simulink model "desaturation"  (R2020b)
settings: Solver=ode15s  StartTime=27585  StopTime=44962.012  MaxStep=0.1  RelTol=1e-8  AbsTol=1e-8
values from neighbouring files (symbols this model uses):
  data = struct()    [config.m]    (also in config6U.m; configSlew.m; mainOffNominal.m = dataFix; statisticalAnalysis.m = dataFix)
undefined symbols (not defined in the file or in its folder): spacecraft
libraries: dspswit3 x1, simulink_extras x1
(part 1 of 2)
settings Model: SimulationMode=accelerator  Creator=pacif  LastModifiedBy=pacif

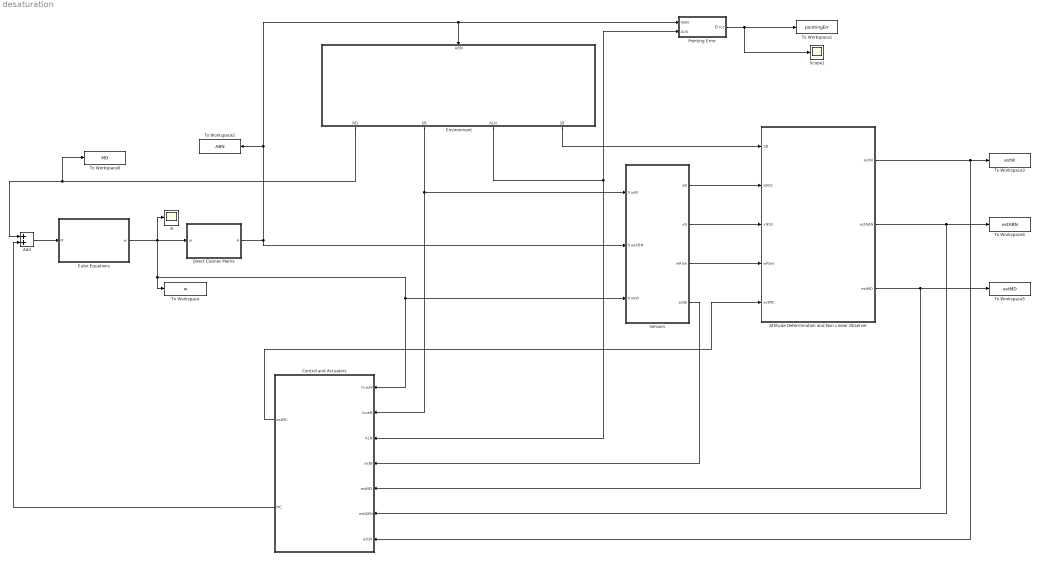
== system desaturation ==
  Add : Sum
  Attitude Determination and Non Linear Observer : Subsystem
  Control and Actuators : Subsystem
  Direct Cosines Matrix : Subsystem
  Environment : Subsystem
  Euler Equations : Subsystem
  Pointing Error : Subsystem
  Scope1 : Scope
  Sensors : Subsystem
  To Workspace : ToWorkspace  VariableName=w  SaveFormat=Timeseries  SampleTime=-1
  To Workspace1 : ToWorkspace  VariableName=pointingErr  SaveFormat=Timeseries  SampleTime=-1
  To Workspace2 : ToWorkspace  VariableName=ABN  SaveFormat=Timeseries  SampleTime=-1
  To Workspace3 : ToWorkspace  VariableName=estW  SaveFormat=Timeseries  SampleTime=-1
  To Workspace4 : ToWorkspace  VariableName=estABN  SaveFormat=Timeseries  SampleTime=-1
  To Workspace5 : ToWorkspace  VariableName=estMD  SaveFormat=Timeseries  SampleTime=-1
  To Workspace6 : ToWorkspace  VariableName=MD  SaveFormat=Timeseries  SampleTime=-1
  w : Scope
  wires:
  Environment/2(bB) -> Sensors/1(trueB), Control and Actuators/2(trueB)
  Add/1 -> Euler Equations/1(M)
  Environment/1(MD) -> To Workspace6/1, Add/1
  Euler Equations/1(w) -> Direct Cosines Matrix/1(w), To Workspace/1, Control and Actuators/1(trueW), Sensors/3(trueW), w/1
  Direct Cosines Matrix/1(A) -> To Workspace2/1, Environment/1(ABN), Pointing Error/1(ABN), Sensors/2(trueABN)
  Environment/3(ALN) -> Pointing Error/2(ALN), Control and Actuators/3(ALN)
  Control and Actuators/2(MC) -> Add/2
  Sensors/4(estB) -> Control and Actuators/4(estB)
  Control and Actuators/1(estMC) -> Attitude Determination and Non Linear Observer/5(estMC)
  Environment/4(SB) -> Attitude Determination and Non Linear Observer/1(SB)
  Attitude Determination and Non Linear Observer/2(estABN) -> Control and Actuators/6(estABN), To Workspace4/1
  Attitude Determination and Non Linear Observer/3(estMD) -> Control and Actuators/5(estMD), To Workspace5/1
  Pointing Error/1(Error) -> Scope1/1, To Workspace1/1
  Sensors/1(sB) -> Attitude Determination and Non Linear Observer/2(sBSS)
  Sensors/2(vN) -> Attitude Determination and Non Linear Observer/3(vNSS)
  Sensors/3(wRaw) -> Attitude Determination and Non Linear Observer/4(wRaw)
  Attitude Determination and Non Linear Observer/1(estW) -> Control and Actuators/7(estW), To Workspace3/1

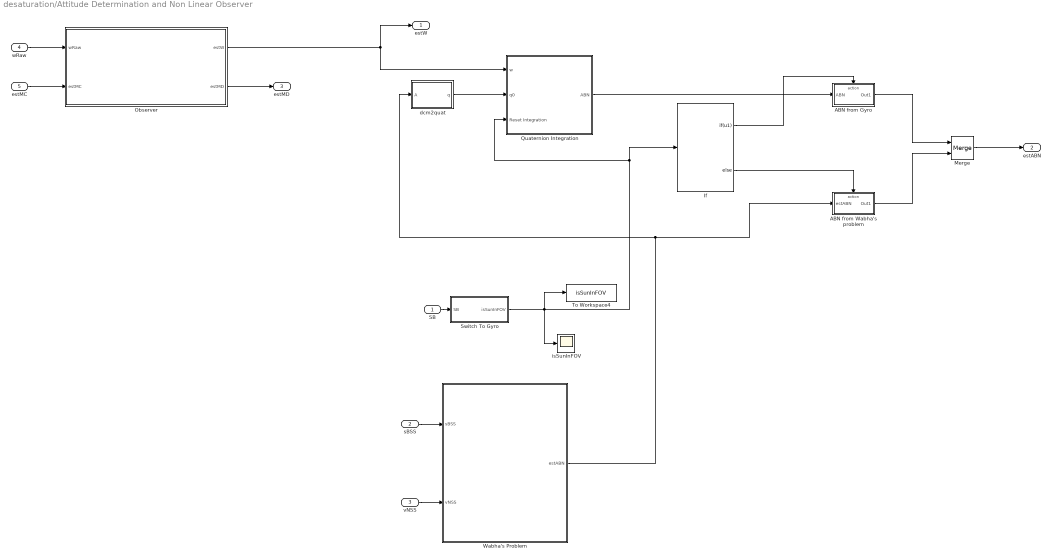
== system desaturation/Attitude Determination and Non Linear Observer ==
  SB : Inport
  sBSS : Inport  Port=2
  vNSS : Inport  Port=3
  wRaw : Inport  Port=4
  estMC : Inport  Port=5
  ABN from Gyro : Subsystem  TreatAsAtomicUnit=on
  ABN from Wabha's problem : Subsystem  TreatAsAtomicUnit=on
  If : If  IfExpression=u1
  Merge : Merge
  Observer : Subsystem
  "Quaternion Integration " : Subsystem
  Switch To Gyro : Subsystem
  To Workspace4 : ToWorkspace  VariableName=isSunInFOV  SaveFormat=Timeseries  SampleTime=-1
  Wabha's Problem : MATLAB Function  TreatAsAtomicUnit=on
  dcm2quat : MATLAB Function  TreatAsAtomicUnit=on
  isSunInFOV : Scope
  estW : Outport
  estABN : Outport  Port=2
  estMD : Outport  Port=3
  wires:
  wRaw/1 -> Observer/1(wRaw)
  SB/1 -> Switch To Gyro/1(SB)
  ABN from Wabha's problem/1(Out1) -> Merge/2
  Merge/1 -> estABN/1
  If/1 -> ABN from Gyro/Action
  If/2 -> ABN from Wabha's problem/Action
  ABN from Gyro/1(Out1) -> Merge/1
  vNSS/1 -> Wabha's Problem/2(vNSS)
  sBSS/1 -> Wabha's Problem/1(sBSS)
  estMC/1 -> Observer/2(estMC)
  Observer/2(estMD) -> estMD/1
  "Quaternion Integration "/1(ABN) -> ABN from Gyro/1(ABN)
  dcm2quat/1(q) -> "Quaternion Integration "/2(q0)
  Switch To Gyro/1(isSunInFOV) -> To Workspace4/1, If/1, "Quaternion Integration "/3(Reset Integration), isSunInFOV/1
  Observer/1(estW) -> "Quaternion Integration "/1(w), estW/1
  Wabha's Problem/1(estABN) -> dcm2quat/1(A), ABN from Wabha's problem/1(estABN)

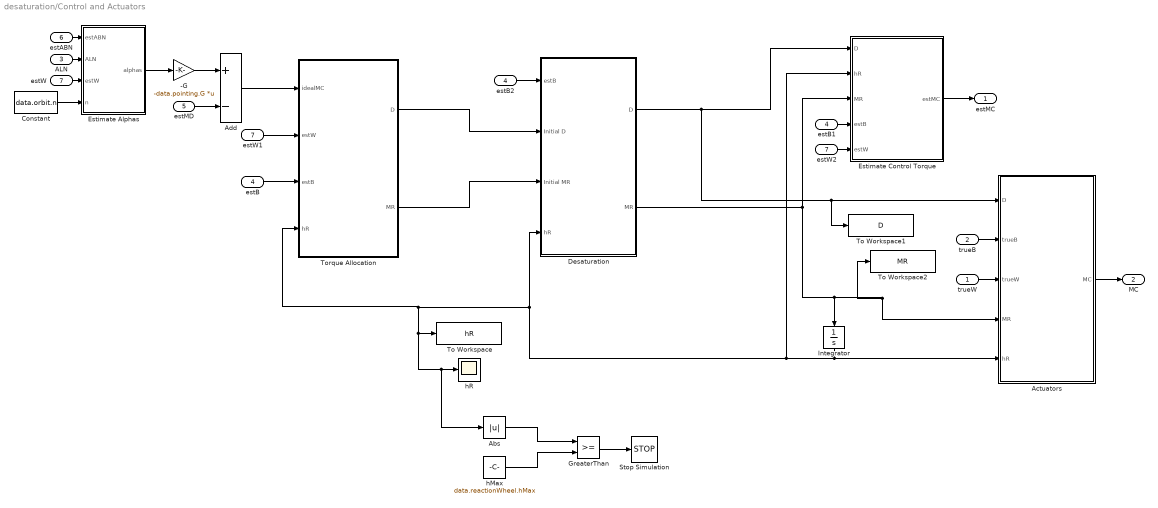
== system desaturation/Control and Actuators ==
  trueW : Inport
  trueB : Inport  Port=2
  ALN : Inport  Port=3
  estB : Inport  Port=4
  estMD : Inport  Port=5
  estABN : Inport  Port=6
  estW : Inport  Port=7
  -G : Gain  Gain=-data.pointing.G  Multiplication=Matrix(K*u) (u vector)
  Abs : Abs
  Actuators : Subsystem
  Add : Sum  Inputs=+-
  Constant : Constant  Value=data.orbit.n
  Desaturation : Subsystem
  Estimate Alphas : MATLAB Function  TreatAsAtomicUnit=on
  Estimate Control Torque : Subsystem
  GreaterThan : RelationalOperator  OutDataTypeStr=boolean  RndMeth=Simplest
  Integrator : Integrator  InitialCondition=data.reactionWheel.h0
  Stop Simulation : Stop
  To Workspace : ToWorkspace  VariableName=hR  SaveFormat=Timeseries  SampleTime=-1
  To Workspace1 : ToWorkspace  VariableName=D  SaveFormat=Timeseries  SampleTime=-1
  To Workspace2 : ToWorkspace  VariableName=MR  SaveFormat=Timeseries  SampleTime=-1
  Torque Allocation : Subsystem
  estB1 : InportShadow  Port=4
  estB2 : InportShadow  Port=4
  estW1 : InportShadow  Port=7
  estW2 : InportShadow  Port=7
  hMax : Constant  Value=data.reactionWheel.hMax
  hR : Scope
  estMC : Outport
  MC : Outport  Port=2
  wires:
  estABN/1 -> Estimate Alphas/1(estABN)
  ALN/1 -> Estimate Alphas/2(ALN)
  Actuators/1(MC) -> MC/1
  trueB/1 -> Actuators/2(trueB)
  trueW/1 -> Actuators/3(trueW)
  Desaturation/2(MR) -> Estimate Control Torque/3(MR), To Workspace2/1, Actuators/4(MR), Integrator/1
  Desaturation/1(D) -> Estimate Control Torque/1(D), Actuators/1(D), To Workspace1/1
  estW/1 -> Estimate Alphas/3(estW)
  estW1/1 -> Torque Allocation/2(estW)
  estB/1 -> Torque Allocation/3(estB)
  estB1/1 -> Estimate Control Torque/4(estB)
  estW2/1 -> Estimate Control Torque/5(estW)
  estMD/1 -> Add/2
  GreaterThan/1 -> Stop Simulation/1
  Abs/1 -> GreaterThan/1
  hMax/1 -> GreaterThan/2
  Constant/1 -> Estimate Alphas/4(n)
  -G/1 -> Add/1
  Add/1 -> Torque Allocation/1(idealMC)
  Estimate Alphas/1(alphas) -> -G/1
  Integrator/1 -> Estimate Control Torque/2(hR), Desaturation/4(hR), Abs/1, hR/1, To Workspace/1, Torque Allocation/4(hR), Actuators/5(hR)
  Estimate Control Torque/1(estMC) -> estMC/1
  estB2/1 -> Desaturation/1(estB)
  Torque Allocation/1(D) -> Desaturation/2(Initial D)
  Torque Allocation/2(MR) -> Desaturation/3(Initial MR)

== system desaturation/Direct Cosines Matrix ==
  w : Inport
  Build 3x3 Matrix : Subsystem
  Constant1 : Constant  Value=0
  Demux1 : Demux  Outputs=3
  Gain{3,5..7} (4 alike) : Gain  Gain=-1
  Integrator : Integrator  InitialCondition=data.ic.dcm
  Orthonormalization : Subsystem
  Product : Product  Multiplication=Matrix(*)
  A : Outport
  wires:
  Demux1/1 -> Build 3x3 Matrix/6(A32), Gain7/1
  Gain5/1 -> Build 3x3 Matrix/4(A12)
  Demux1/3 -> Build 3x3 Matrix/2(A21), Gain5/1
  Product/1 -> Gain3/1
  Build 3x3 Matrix/1(A) -> Product/1  "[w]^"
  Gain6/1 -> Build 3x3 Matrix/3(A31)
  Demux1/2 -> Build 3x3 Matrix/7("A13 "), Gain6/1
  Gain7/1 -> Build 3x3 Matrix/8(A23)
  Orthonormalization/1(A) -> Product/2, A/1
  Gain3/1 -> Integrator/1  "dA/dt"
  w/1 -> Demux1/1
  Integrator/1 -> Orthonormalization/1(A0)  "A"
  Constant1/1 -> Build 3x3 Matrix/1(A11), Build 3x3 Matrix/9(A33), Build 3x3 Matrix/5(A22)

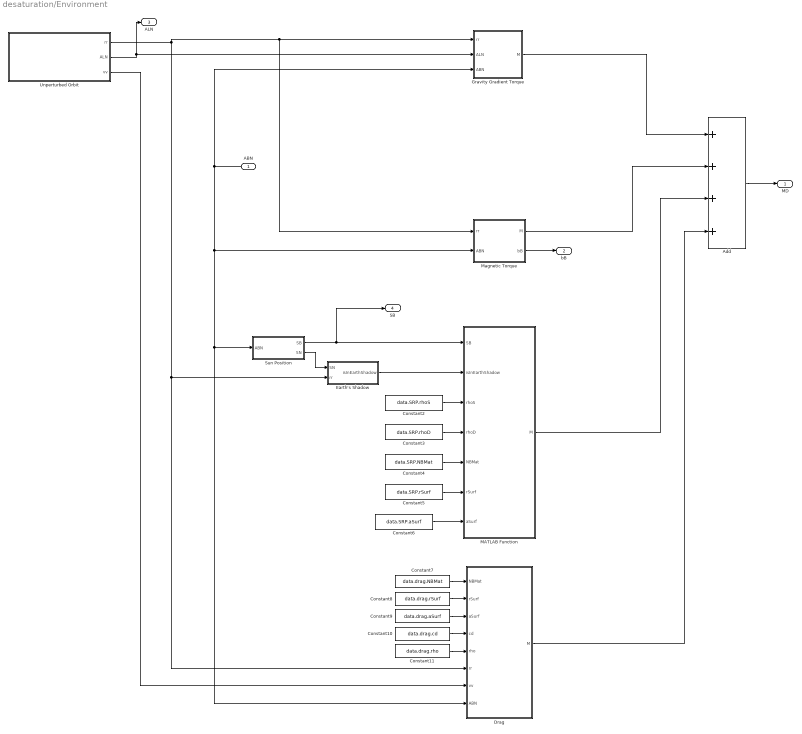
== system desaturation/Environment ==
  ABN : Inport
  Add : Sum  Inputs=++++
  Constant10 : Constant  Value=data.drag.cd
  Constant11 : Constant  Value=data.drag.rho
  Constant2 : Constant  Value=data.SRP.rhoS
  Constant3 : Constant  Value=data.SRP.rhoD
  Constant4 : Constant  Value=data.SRP.NBMat
  Constant5 : Constant  Value=data.SRP.rSurf
  Constant6 : Constant  Value=data.SRP.aSurf
  Constant7 : Constant  Value=data.drag.NBMat
  Constant8 : Constant  Value=data.drag.rSurf
  Constant9 : Constant  Value=data.drag.aSurf
  Drag : MATLAB Function  TreatAsAtomicUnit=on
  Earth's Shadow : Subsystem
  Gravity Gradient Torque : Subsystem
  MATLAB Function : MATLAB Function  TreatAsAtomicUnit=on
  Magnetic Torque : Subsystem
  "Sun Position " : Subsystem
  Unperturbed Orbit : Subsystem
  MD : Outport
  bB : Outport  Port=2
  ALN : Outport  Port=3
  SB : Outport  Port=4
  wires:
  Earth's Shadow/1(isInEarthShadow) -> MATLAB Function/2(isInEarthShadow)
  Constant5/1 -> MATLAB Function/6(rSurf)
  Constant6/1 -> MATLAB Function/7(aSurf)
  Constant3/1 -> MATLAB Function/4(rhoD)
  Constant4/1 -> MATLAB Function/5(NBMat)
  Gravity Gradient Torque/1(M) -> Add/1
  Unperturbed Orbit/1(rr) -> Magnetic Torque/1(rr), Gravity Gradient Torque/1(rr), Earth's Shadow/2(rr), Drag/6(rr)
  MATLAB Function/1(M) -> Add/3
  Constant10/1 -> Drag/4(cd)
  Drag/1(M) -> Add/4
  ABN/1 -> Gravity Gradient Torque/3(ABN), Magnetic Torque/2(ABN), Drag/8(ABN), "Sun Position "/1(ABN)
  Constant7/1 -> Drag/1(NBMat)
  Constant8/1 -> Drag/2(rSurf)
  Constant9/1 -> Drag/3(aSurf)
  Add/1 -> MD/1
  Constant2/1 -> MATLAB Function/3(rhoS)
  Magnetic Torque/1(M) -> Add/2
  Unperturbed Orbit/2(ALN) -> ALN/1, Gravity Gradient Torque/2(ALN)
  Constant11/1 -> Drag/5(rho)
  Unperturbed Orbit/3(vv) -> Drag/7(vv)
  Magnetic Torque/2(bB) -> bB/1
  "Sun Position "/2(SN) -> Earth's Shadow/1(SN)
  "Sun Position "/1(SB) -> SB/1, MATLAB Function/1(SB)

== system desaturation/Euler Equations ==
  M : Inport
  Add : Sum
  Cross Product : Subsystem
  Gain : Gain  Gain=data.sc.invI  Multiplication=Matrix(K*u) (u vector)
  Gain2 : Gain  Gain=data.sc.inertiaMatrix  Multiplication=Matrix(K*u) (u vector)
  Integrator : Integrator  InitialCondition=data.ic.w
  w : Outport
  wires:
  Gain2/1 -> Cross Product/1(a)  "I*w"
  Cross Product/1(c) -> Add/2  "I*w x w = -w x I*w"
  M/1 -> Add/1
  Integrator/1 -> Cross Product/2(b), Gain2/1, w/1  "w"
  Gain/1 -> Integrator/1  "dw"
  Add/1 -> Gain/1

== system desaturation/Pointing Error ==
  ABN : Inport
  ALN : Inport  Port=2
  Acos : Trigonometry  Operator=acos
  Product : Product  Multiplication=Matrix(*)
  Radians to Degrees : simulink_extras/Transformations/Radians to Degrees
  Selector : Selector  NumberOfDimensions=2  InputPortWidth=3  IndexOptions=Index vector (dialog),Index vector (dialog)  Indices=1,1  OutputSizes=1,1
  Transpose : Math  Operator=transpose  SaturateOnIntegerOverflow=on
  Error : Outport
  wires:
  Radians to Degrees/1 -> Error/1
  ABN/1 -> Product/1
  ALN/1 -> Transpose/1
  Transpose/1 -> Product/2
  Product/1 -> Selector/1
  Selector/1 -> Acos/1
  Acos/1 -> Radians to Degrees/1

== system desaturation/Sensors ==
  trueB : Inport
  trueABN : Inport  Port=2
  trueW : Inport  Port=3
  Add3 : Sum  Inputs=+-
  Gyro Error : Scope
  Gyroscope : Subsystem
  Magnetometer : Subsystem
  Star Sensor : Subsystem
  sB : Outport
  vN : Outport  Port=2
  wRaw : Outport  Port=3
  estB : Outport  Port=4
  wires:
  Magnetometer/1(estB) -> estB/1
  Add3/1 -> Gyro Error/1
  trueABN/1 -> Star Sensor/1(ABN)
  Star Sensor/1(sB) -> sB/1
  Star Sensor/2(vN) -> vN/1
  Gyroscope/1(wRaw) -> wRaw/1, Add3/2
  trueB/1 -> Magnetometer/1(B)
  trueW/1 -> Add3/1, Gyroscope/1(trueW)

== system desaturation/Attitude Determination and Non Linear Observer/ABN from Gyro ==
  ABN : Inport
  Action Port : ActionPort  ActionPortLabel=if(u1)
  Out1 : Outport
  wires:
  ABN/1 -> Out1/1

== system desaturation/Attitude Determination and Non Linear Observer/ABN from Wabha's problem ==
  estABN : Inport
  Action Port : ActionPort  ActionPortLabel=else
  Out1 : Outport
  wires:
  estABN/1 -> Out1/1

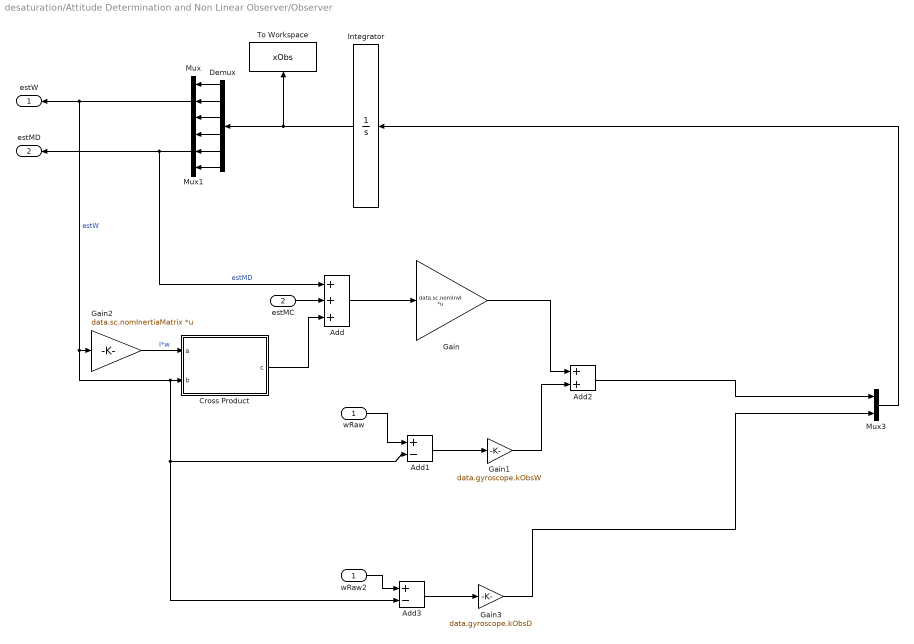
== system desaturation/Attitude Determination and Non Linear Observer/Observer ==
  wRaw : Inport
  estMC : Inport  Port=2
  Add : Sum  Inputs=+++
  Add1 : Sum  Inputs=+-
  Add2 : Sum
  Add3 : Sum  Inputs=+-
  Cross Product : Subsystem
  Demux : Demux  Outputs=6
  Gain : Gain  Gain=data.sc.nomInvI  Multiplication=Matrix(K*u) (u vector)
  Gain1 : Gain  Gain=data.gyroscope.kObsW
  Gain2 : Gain  Gain=data.sc.nomInertiaMatrix  Multiplication=Matrix(K*u) (u vector)
  Gain3 : Gain  Gain=data.gyroscope.kObsD
  Integrator : Integrator  InitialCondition=data.gyroscope.xObs0
  Mux : Mux  Inputs=3
  Mux1 : Mux  Inputs=3
  Mux3 : Mux  Inputs=2
  To Workspace : ToWorkspace  VariableName=xObs  SaveFormat=Timeseries  SampleTime=-1
  wRaw2 : InportShadow
  estW : Outport
  estMD : Outport  Port=2
  wires:
  Mux3/1 -> Integrator/1
  Integrator/1 -> Demux/1, To Workspace/1
  estMC/1 -> Add/2
  Demux/1 -> Mux/1
  Demux/2 -> Mux/2
  Demux/3 -> Mux/3
  Demux/5 -> Mux1/2
  Demux/4 -> Mux1/1
  Demux/6 -> Mux1/3
  Mux1/1 -> Add/1, estMD/1  "estMD"
  Cross Product/1(c) -> Add/3
  Add/1 -> Gain/1
  Gain2/1 -> Cross Product/1(a)  "I*w"
  Gain/1 -> Add2/1
  wRaw/1 -> Add1/1
  Add1/1 -> Gain1/1
  Gain1/1 -> Add2/2
  Add2/1 -> Mux3/1
  Add3/1 -> Gain3/1
  Mux/1 -> Add3/2, Add1/2, Cross Product/2(b), Gain2/1, estW/1  "estW"
  Gain3/1 -> Mux3/2
  wRaw2/1 -> Add3/1

== system desaturation/Attitude Determination and Non Linear Observer/Quaternion Integration  ==
  w : Inport
  q0 : Inport  Port=2
  Reset Integration : Inport  Port=3
  Gain : Gain  Gain=0.5
  Integrator : Integrator  ExternalReset=either  InitialConditionSource=external  InitialCondition=spacecraft.q0
  M1 : Subsystem
  M2 : Subsystem
  "Normalization " : Subsystem
  Product : Product  Multiplication=Matrix(*)
  ABN : Outport
  wires:
  w/1 -> M1/1(w)
  M1/1(M1) -> Gain/1
  Gain/1 -> Product/1
  Product/1 -> Integrator/1  "q_dot"
  Integrator/1 -> "Normalization "/1("q ")  "q"
  M2/1("M2 ") -> ABN/1
  "Normalization "/1(qNormalized) -> M2/1(q), Product/2
  Reset Integration/1 -> Integrator/2
  q0/1 -> Integrator/3

== system desaturation/Attitude Determination and Non Linear Observer/Switch To Gyro ==
  SB : Inport
  ASB : Gain  Gain=data.starSensor.ABS'  Multiplication=Matrix(K*u) (u vector)
  Acos : Trigonometry  Operator=acos
  FOV/2 : Constant  Value=data.starSensor.FOV/2
  Less Than : RelationalOperator  Operator=<  OutDataTypeStr=boolean  ZeroCross=off  RndMeth=Simplest
  Selector : Selector  InputPortWidth=3  IndexOptions=Index vector (dialog)  Indices=[3]  OutputSizes=1
  isSunInFOV : Outport
  wires:
  ASB/1 -> Selector/1
  FOV/2/1 -> Less Than/2
  Acos/1 -> Less Than/1
  SB/1 -> ASB/1
  Selector/1 -> Acos/1
  Less Than/1 -> isSunInFOV/1

== system desaturation/Control and Actuators/Actuators ==
  D : Inport
  trueB : Inport  Port=2
  trueW : Inport  Port=3
  MR : Inport  Port=4
  hR : Inport  Port=5
  Add : Sum
  Add1 : Sum
  Cross Product : Subsystem
  Cross Product1 : Subsystem
  Gain : Gain  Gain=-1
  Product : Product
  Product1 : Product
  Reaction Wheel Axis : Constant  Value=data.reactionWheel.axis
  MC : Outport
  wires:
  D/1 -> Cross Product/1(a)
  trueB/1 -> Cross Product/2(b)
  Add/1 -> MC/1
  Cross Product/1(c) -> Add/1
  Gain/1 -> Add/2
  Add1/1 -> Gain/1
  Cross Product1/1(c) -> Add1/1
  trueW/1 -> Cross Product1/1(a)
  Product/1 -> Cross Product1/2(b)
  MR/1 -> Product1/2
  hR/1 -> Product/1
  Reaction Wheel Axis/1 -> Product1/1, Product/2
  Product1/1 -> Add1/2

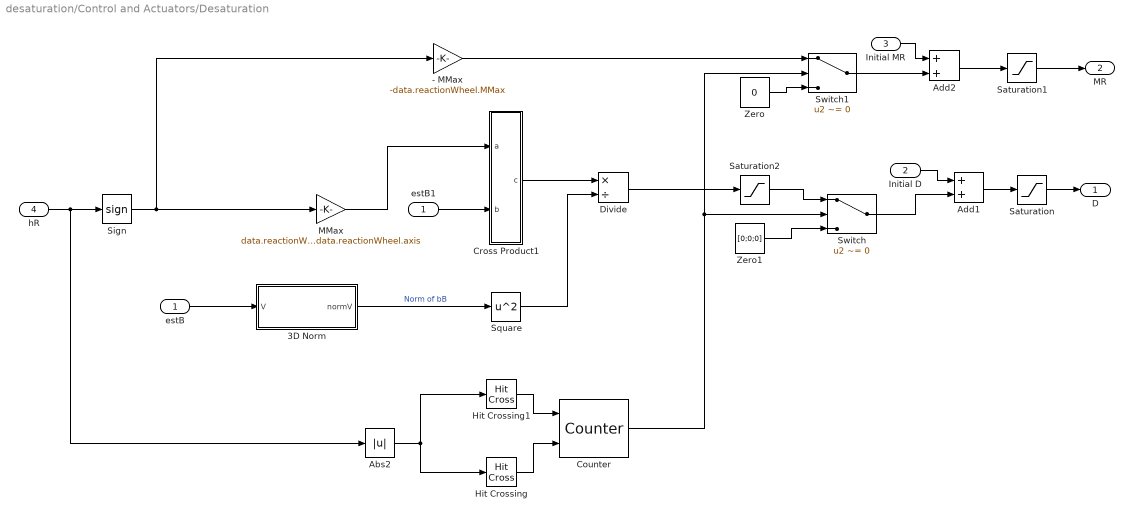
== system desaturation/Control and Actuators/Desaturation ==
  estB : Inport
  Initial D : Inport  Port=2
  Initial MR : Inport  Port=3
  hR : Inport  Port=4
  - MMax : Gain  Gain=-data.reactionWheel.MMax
  3D Norm : Subsystem
  Abs2 : Abs
  Add1 : Sum
  Add2 : Sum
  Counter : dspswit3/Counter  Direction=Up  CountEvent=Rising edge  CounterSize=User defined  MaxCount=255  InitialCount=0  Output=Count  HitValue=32  ResetInput=on  SamplesPerFrame=1  Ts=1  CntDtype=double  HitDtype=Logical
  Cross Product1 : Subsystem
  Divide : Product  Inputs=*/
  Hit Crossing : HitCross  HitCrossingOffset=data.desaturation.hLow  HitCrossingDirection=falling
  Hit Crossing1 : HitCross  HitCrossingOffset=data.desaturation.hUp  HitCrossingDirection=rising
  MMax : Gain  Gain=data.reactionWheel.MMax*data.reactionWheel.axis
  Saturation : Saturate  UpperLimit=data.magnetorquer.DMax  LowerLimit=-data.magnetorquer.DMax  LinearizeAsGain=off
  Saturation1 : Saturate  UpperLimit=data.reactionWheel.MMax  LowerLimit=-data.reactionWheel.MMax
  Saturation2 : Saturate  UpperLimit=data.magnetorquer.DMax  LowerLimit=-data.magnetorquer.DMax  LinearizeAsGain=off
  Sign : Signum
  Square : Math  Operator=square  SaturateOnIntegerOverflow=on
  Switch : Switch  Criteria=u2 ~= 0
  Switch1 : Switch  Criteria=u2 ~= 0
  Zero : Constant  Value=0  OutDataTypeStr=Inherit: Inherit via back propagation
  Zero1 : Constant  Value=[0;0;0]  OutDataTypeStr=Inherit: Inherit via back propagation
  estB1 : InportShadow
  D : Outport
  MR : Outport  Port=2
  wires:
  3D Norm/1(normV) -> Square/1  "Norm of bB"
  - MMax/1 -> Switch1/1
  Square/1 -> Divide/2
  Cross Product1/1(c) -> Divide/1
  Divide/1 -> Saturation2/1
  MMax/1 -> Cross Product1/1(a)
  Sign/1 -> MMax/1, - MMax/1
  hR/1 -> Sign/1, Abs2/1
  estB/1 -> 3D Norm/1(V)
  Add1/1 -> Saturation/1
  Add2/1 -> Saturation1/1
  Switch1/1 -> Add2/2
  Zero1/1 -> Switch/3
  Zero/1 -> Switch1/3
  Counter/1 -> Switch/2, Switch1/2
  Hit Crossing/1 -> Counter/2
  Switch/1 -> Add1/2
  Abs2/1 -> Hit Crossing/1, Hit Crossing1/1
  Hit Crossing1/1 -> Counter/1
  Initial D/1 -> Add1/1
  Initial MR/1 -> Add2/1
  Saturation1/1 -> MR/1
  Saturation/1 -> D/1
  estB1/1 -> Cross Product1/2(b)
  Saturation2/1 -> Switch/1

== system desaturation/Control and Actuators/Estimate Control Torque ==
  D : Inport
  hR : Inport  Port=2
  MR : Inport  Port=3
  estB : Inport  Port=4
  estW : Inport  Port=5
  Add : Sum  Inputs=+--
  Cross Product : Subsystem
  Cross Product1 : Subsystem
  Product : Product
  Product1 : Product
  RW Axis : Constant  Value=data.reactionWheel.axis
  RW Axis1 : Constant  Value=data.reactionWheel.axis
  estMC : Outport
  wires:
  D/1 -> Cross Product/1(a)
  estB/1 -> Cross Product/2(b)
  Add/1 -> estMC/1
  Cross Product/1(c) -> Add/1
  RW Axis/1 -> Product/1
  MR/1 -> Product/2
  Product/1 -> Add/2
  Cross Product1/1(c) -> Add/3
  estW/1 -> Cross Product1/1(a)
  hR/1 -> Product1/2
  RW Axis1/1 -> Product1/1
  Product1/1 -> Cross Product1/2(b)

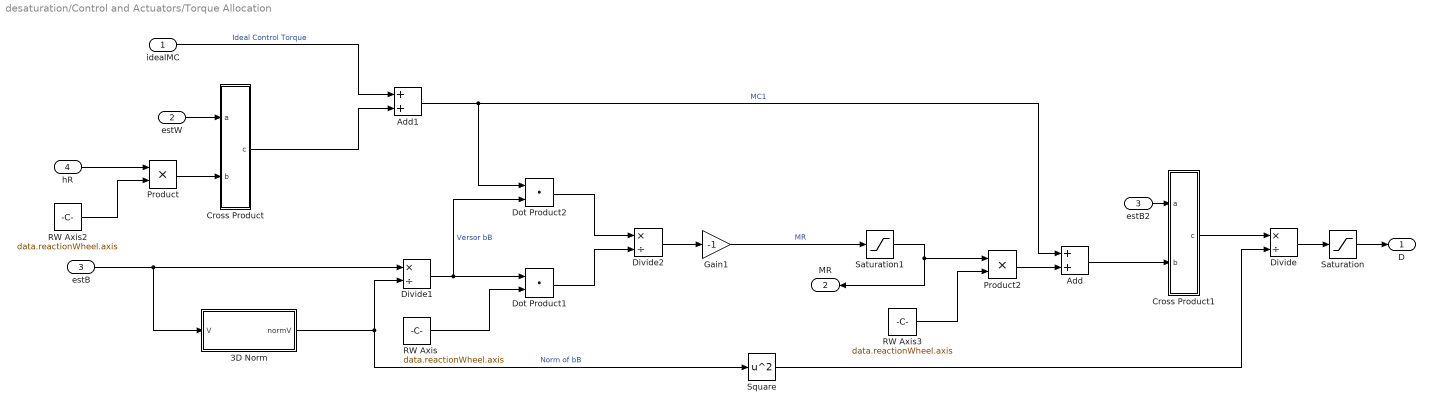
== system desaturation/Control and Actuators/Torque Allocation ==
  idealMC : Inport
  estW : Inport  Port=2
  estB : Inport  Port=3
  hR : Inport  Port=4
  3D Norm : Subsystem
  Add : Sum
  Add1 : Sum
  Cross Product : Subsystem
  Cross Product1 : Subsystem
  Divide : Product  Inputs=*/
  Divide1 : Product  Inputs=*/
  Divide2 : Product  Inputs=*/
  Dot Product1 : DotProduct  InputSameDT=on  OutDataTypeStr=Inherit: Inherit via internal rule
  Dot Product2 : DotProduct  InputSameDT=on  OutDataTypeStr=Inherit: Inherit via internal rule
  Gain1 : Gain  Gain=-1
  Product : Product
  Product2 : Product
  RW Axis : Constant  Value=data.reactionWheel.axis
  RW Axis2 : Constant  Value=data.reactionWheel.axis
  RW Axis3 : Constant  Value=data.reactionWheel.axis
  Saturation : Saturate  UpperLimit=data.magnetorquer.DMax  LowerLimit=-data.magnetorquer.DMax  LinearizeAsGain=off
  Saturation1 : Saturate  UpperLimit=data.reactionWheel.MMax  LowerLimit=-data.reactionWheel.MMax
  Square : Math  Operator=square  SaturateOnIntegerOverflow=on
  estB2 : InportShadow  Port=3
  D : Outport
  MR : Outport  Port=2
  wires:
  Cross Product/1(c) -> Add1/2
  idealMC/1 -> Add1/1  "Ideal Control Torque"
  Product/1 -> Cross Product/2(b)
  hR/1 -> Product/1
  estW/1 -> Cross Product/1(a)
  Add1/1 -> Dot Product2/1, Add/1  "MC1"
  estB/1 -> Divide1/1, 3D Norm/1(V)
  3D Norm/1(normV) -> Square/1, Divide1/2  "Norm of bB"
  Divide1/1 -> Dot Product2/2, Dot Product1/1  "Versor bB"
  RW Axis/1 -> Dot Product1/2
  Dot Product2/1 -> Divide2/1
  Dot Product1/1 -> Divide2/2
  Divide2/1 -> Gain1/1
  Gain1/1 -> Saturation1/1  "MR"
  Saturation1/1 -> Product2/1, MR/1
  Product2/1 -> Add/2
  RW Axis2/1 -> Product/2
  RW Axis3/1 -> Product2/2
  Add/1 -> Cross Product1/2(b)
  estB2/1 -> Cross Product1/1(a)
  Cross Product1/1(c) -> Divide/1
  Square/1 -> Divide/2
  Saturation/1 -> D/1
  Divide/1 -> Saturation/1

== system desaturation/Direct Cosines Matrix/Build 3x3 Matrix ==
  A11 : Inport
  A21 : Inport  Port=2
  A31 : Inport  Port=3
  A12 : Inport  Port=4
  A22 : Inport  Port=5
  A32 : Inport  Port=6
  "A13 " : Inport  Port=7
  A23 : Inport  Port=8
  A33 : Inport  Port=9
  Mux : Mux  Inputs=3
  Mux1 : Mux  Inputs=3
  Mux2 : Mux  Inputs=3
  Vector Concatenate : Concatenate  NumInputs=3  Mode=Multidimensional array  ConcatenateDimension=2
  A : Outport
  wires:
  A21/1 -> Mux/2
  A23/1 -> Mux2/2
  "A13 "/1 -> Mux2/1
  A11/1 -> Mux/1
  Vector Concatenate/1 -> A/1
  A31/1 -> Mux/3
  A12/1 -> Mux1/1
  A22/1 -> Mux1/2
  Mux2/1 -> Vector Concatenate/3
  Mux1/1 -> Vector Concatenate/2
  Mux/1 -> Vector Concatenate/1
  A33/1 -> Mux2/3
  A32/1 -> Mux1/3

== system desaturation/Direct Cosines Matrix/Orthonormalization ==
  A0 : Inport
  Add : Sum  Inputs=+-
  Gain : Gain  Gain=1.5
  Gain1 : Gain  Gain=0.5
  Product : Product  Inputs=3  Multiplication=Matrix(*)
  Transpose : Math  Operator=transpose  SaturateOnIntegerOverflow=on
  A : Outport
  wires:
  Add/1 -> A/1
  A0/1 -> Product/3, Transpose/1, Product/1, Gain/1
  Gain1/1 -> Add/2
  Gain/1 -> Add/1
  Transpose/1 -> Product/2
  Product/1 -> Gain1/1

== system desaturation/Environment/Earth's Shadow ==
  SN : Inport
  rr : Inport  Port=2
  1 AU : Constant  Value=1.496e8
  3D Norm : Subsystem
  Acos : Trigonometry  Operator=acos
  Acos1 : Trigonometry  Operator=acos
  Acos2 : Trigonometry  Operator=acos
  Add : Sum
  Divide : Product  Inputs=*/
  Divide1 : Product  Inputs=*/
  Divide2 : Product  Inputs=*/
  Dot Product : DotProduct  InputSameDT=on  OutDataTypeStr=Inherit: Inherit via internal rule
  Earth's Radius : Constant  Value=6371
  GreaterThan : RelationalOperator  Operator=>  OutDataTypeStr=boolean  RndMeth=Simplest
  isInEarthShadow : Outport
  wires:
  SN/1 -> Dot Product/2
  GreaterThan/1 -> isInEarthShadow/1
  Add/1 -> GreaterThan/2
  Acos/1 -> GreaterThan/1
  Acos2/1 -> Add/2
  Acos1/1 -> Add/1
  rr/1 -> 3D Norm/1(V), Divide/1
  3D Norm/1(normV) -> Divide1/2, Divide/2
  Divide/1 -> Dot Product/1
  Dot Product/1 -> Acos/1
  Earth's Radius/1 -> Divide1/1, Divide2/1
  Divide1/1 -> Acos1/1
  Divide2/1 -> Acos2/1
  1 AU/1 -> Divide2/2

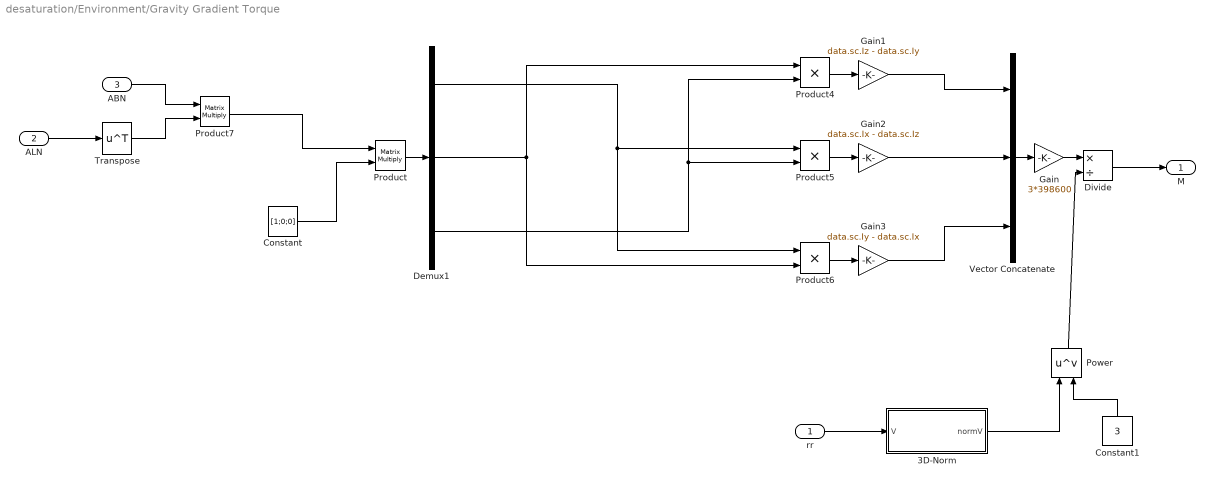
== system desaturation/Environment/Gravity Gradient Torque ==
  rr : Inport
  ALN : Inport  Port=2
  ABN : Inport  Port=3
  3D-Norm : Subsystem
  Constant : Constant  Value=[1;0;0]  VectorParams1D=off
  Constant1 : Constant  Value=3
  Demux1 : Demux  Outputs=3
  Divide : Product  Inputs=*/
  Gain : Gain  Gain=3*398600
  Gain1 : Gain  Gain=data.sc.Iz - data.sc.Iy
  Gain2 : Gain  Gain=data.sc.Ix - data.sc.Iz
  Gain3 : Gain  Gain=data.sc.Iy - data.sc.Ix
  Power : Math  Operator=pow  SaturateOnIntegerOverflow=on
  Product : Product  Multiplication=Matrix(*)
  Product4 : Product
  Product5 : Product
  Product6 : Product
  Product7 : Product  Multiplication=Matrix(*)
  Transpose : Math  Operator=transpose  SaturateOnIntegerOverflow=on
  Vector Concatenate : Concatenate  NumInputs=3
  M : Outport
  wires:
  Constant/1 -> Product/2
  Gain3/1 -> Vector Concatenate/3
  Gain1/1 -> Vector Concatenate/1
  Gain2/1 -> Vector Concatenate/2
  Vector Concatenate/1 -> Gain/1
  Constant1/1 -> Power/2
  Power/1 -> Divide/2
  Gain/1 -> Divide/1
  Product/1 -> Demux1/1
  Product4/1 -> Gain1/1
  Product5/1 -> Gain2/1
  Product6/1 -> Gain3/1
  Demux1/1 -> Product6/1, Product5/1
  Demux1/2 -> Product6/2, Product4/1
  Demux1/3 -> Product5/2, Product4/2
  Divide/1 -> M/1
  rr/1 -> 3D-Norm/1(V)
  3D-Norm/1(normV) -> Power/1
  ALN/1 -> Transpose/1
  Product7/1 -> Product/1
  ABN/1 -> Product7/1
  Transpose/1 -> Product7/2

== system desaturation/Environment/Magnetic Torque ==
  rr : Inport
  ABN : Inport  Port=2
  Cross Product : Subsystem
  Product : Product  Multiplication=Matrix(*)
  Subsystem : Subsystem
  m : Constant  Value=data.magneticTorque.m
  M : Outport
  bB : Outport  Port=2
  wires:
  rr/1 -> Subsystem/1(rr)
  ABN/1 -> Product/1
  Subsystem/1(bN) -> Product/2
  m/1 -> Cross Product/1(a)
  Product/1 -> Cross Product/2(b), bB/1
  Cross Product/1(c) -> M/1

== system desaturation/Environment/Sun Position  ==
  ABN : Inport
  Clock : Clock
  Cos : Trigonometry  Operator=cos
  Gain1 : Gain  Gain=2*pi/365/24/3600
  Gain2 : Gain  Gain=cos(23.45*pi/180)
  Gain3 : Gain  Gain=sin(23.45*pi/180)
  Mux : Mux  Inputs=3
  Product : Product  Multiplication=Matrix(*)
  Sin : Trigonometry
  Sin1 : Trigonometry
  SB : Outport
  SN : Outport  Port=2
  wires:
  Clock/1 -> Gain1/1
  Mux/1 -> SN/1, Product/2  "SN"
  Gain2/1 -> Mux/2
  Gain3/1 -> Mux/3
  Cos/1 -> Mux/1
  Sin1/1 -> Gain3/1
  Sin/1 -> Gain2/1
  Gain1/1 -> Sin/1, Sin1/1, Cos/1
  ABN/1 -> Product/1
  Product/1 -> SB/1

== system desaturation/Environment/Unperturbed Orbit ==
  Integrator : Integrator  InitialCondition=data.ic.th
  Subsystem : Subsystem
  Subsystem1 : Subsystem
  Subsystem2 : Subsystem
  Subsystem3 : Subsystem
  To Workspace : ToWorkspace  VariableName=theta  SaveFormat=Timeseries  SampleTime=-1
  rr : Outport
  ALN : Outport  Port=2
  vv : Outport  Port=3
  wires:
  Integrator/1 -> Subsystem2/1(theta), Subsystem1/1(theta), Subsystem3/1(theta), To Workspace/1, Subsystem/1(theta)
  Subsystem2/1(rr) -> rr/1
  Subsystem/1(theta_dot) -> Integrator/1
  Subsystem1/1(ALN) -> ALN/1
  Subsystem3/1(vv) -> vv/1

== system desaturation/Euler Equations/Cross Product ==
  a : Inport
  b : Inport  Port=2
  Add : Sum  Inputs=+-
  Add1 : Sum  Inputs=+-
  Add2 : Sum  Inputs=+-
  Demux : Demux  Outputs=3
  Demux1 : Demux  Outputs=3
  Product{,1..5} (6 alike) : Product
  Vector Concatenate : Concatenate  NumInputs=3
  c : Outport
  wires:
  Demux1/1 -> Product2/2, Product5/2  "Bx"
  Product2/1 -> Add1/1
  Vector Concatenate/1 -> c/1
  Add/1 -> Vector Concatenate/1
  Product3/1 -> Add1/2
  Product1/1 -> Add/2
  Product4/1 -> Add2/1
  Product/1 -> Add/1
  Demux/1 -> Product3/1, Product4/1  "Ax"
  Product5/1 -> Add2/2
  Demux/3 -> Product2/1, Product1/1  "Az"
  b/1 -> Demux1/1
  a/1 -> Demux/1
  Add2/1 -> Vector Concatenate/3
  Demux/2 -> Product5/1, Product/1  "Ay"
  Demux1/3 -> Product/2, Product3/2  "Bz"
  Demux1/2 -> Product4/2, Product1/2  "By"
  Add1/1 -> Vector Concatenate/2

== system desaturation/Sensors/Gyroscope ==
  trueW : Inport
  Add : Sum
  Add1 : Sum
  Integrator : Integrator  InitialCondition=data.gyroscope.b0
  Random Number : RandomNumber  Variance=data.gyroscope.sigmaN^2*[1;1;1]  Seed=[2323; 3445;34]  SampleTime=data.gyroscope.sampleTime
  Random Number1 : RandomNumber  Variance=data.gyroscope.sigmaB^2*[1;1;1]  Seed=[34432; 345456;1087]  SampleTime=data.gyroscope.sampleTime
  To Workspace : ToWorkspace  VariableName=bGyro  SaveFormat=Timeseries  SampleTime=-1
  Zero-Order Hold : ZeroOrderHold  SampleTime=data.gyroscope.sampleTime
  wRaw : Outport
  wires:
  Zero-Order Hold/1 -> wRaw/1
  Add/1 -> Zero-Order Hold/1
  Random Number/1 -> Add1/1
  Add1/1 -> Add/2
  trueW/1 -> Add/1
  Integrator/1 -> To Workspace/1, Add1/2
  Random Number1/1 -> Integrator/1

== system desaturation/Sensors/Magnetometer ==
  B : Inport
  Add : Sum
  Multiply : Gain  Gain=data.magnetometer.nonOrthogonality  Multiplication=Matrix(K*u) (u vector)
  Random Number1 : RandomNumber  Variance=(data.magnetometer.sigma)^2*[1;1;1]  Seed=randi(1e5,3,1)  SampleTime=data.magnetometer.sampleTime
  Zero-Order Hold : ZeroOrderHold  SampleTime=data.magnetometer.sampleTime
  estB : Outport
  wires:
  Random Number1/1 -> Add/2
  Add/1 -> Zero-Order Hold/1
  B/1 -> Add/1
  Zero-Order Hold/1 -> Multiply/1
  Multiply/1 -> estB/1

== system desaturation/Sensors/Star Sensor ==
  ABN : Inport
  Constant : Constant  Value=data.starSensor.ABS
  Constant1 : Constant  Value=data.starSensor.FOV
  MATLAB Function : MATLAB Function  TreatAsAtomicUnit=on
  Random Number : RandomNumber  Variance=data.starSensor.sigmaCross^2*ones(2*data.starSensor.NStars,1)  Seed=randi(1e5,2*data.starSensor.NStars,1)  SampleTime=data.starSensor.sampleTime  VectorParams1D=off
  Random Number1 : RandomNumber  Variance=data.starSensor.sigmaRoll^2*ones(data.starSensor.NStars,1)  Seed=randi(1e5,data.starSensor.NStars,1)  SampleTime=data.starSensor.sampleTime
  Uniform Random Number : UniformRandomNumber  Seed=randi(1e5,data.starSensor.NStars*2,1)  SampleTime=data.starSensor.sampleTime
  Zero-Order Hold3 : ZeroOrderHold  SampleTime=data.starSensor.sampleTime
  sB : Outport
  vN : Outport  Port=2
  wires:
  Constant/1 -> MATLAB Function/6(ABS)
  Constant1/1 -> MATLAB Function/4(FOV)
  ABN/1 -> Zero-Order Hold3/1
  MATLAB Function/1(sB) -> sB/1
  MATLAB Function/2(vN) -> vN/1
  Random Number/1 -> MATLAB Function/1(errCross)
  Zero-Order Hold3/1 -> MATLAB Function/5(ABN)
  Random Number1/1 -> MATLAB Function/2(errRoll)
  Uniform Random Number/1 -> MATLAB Function/3(randUniform)

== system desaturation/Attitude Determination and Non Linear Observer/Observer/Cross Product ==
  a : Inport
  b : Inport  Port=2
  Add : Sum  Inputs=+-
  Add1 : Sum  Inputs=+-
  Add2 : Sum  Inputs=+-
  Demux : Demux  Outputs=3
  Demux1 : Demux  Outputs=3
  Product{,1..5} (6 alike) : Product
  Vector Concatenate : Concatenate  NumInputs=3
  c : Outport
  wires:
  Demux1/1 -> Product2/2, Product5/2  "Bx"
  Product2/1 -> Add1/1
  Vector Concatenate/1 -> c/1
  Add/1 -> Vector Concatenate/1
  Product3/1 -> Add1/2
  Product1/1 -> Add/2
  Product4/1 -> Add2/1
  Product/1 -> Add/1
  Demux/1 -> Product3/1, Product4/1  "Ax"
  Product5/1 -> Add2/2
  Demux/3 -> Product2/1, Product1/1  "Az"
  b/1 -> Demux1/1
  a/1 -> Demux/1
  Add2/1 -> Vector Concatenate/3
  Demux/2 -> Product5/1, Product/1  "Ay"
  Demux1/3 -> Product/2, Product3/2  "Bz"
  Demux1/2 -> Product4/2, Product1/2  "By"
  Add1/1 -> Vector Concatenate/2

== system desaturation/Attitude Determination and Non Linear Observer/Quaternion Integration /M1 ==
  w : Inport
  Build 4x4 Matrix1 : Subsystem
  Constant{1..4} (4 alike) : Constant  Value=0
  Demux1 : Demux  Outputs=3
  Gain{3..8} (6 alike) : Gain  Gain=-1
  M1 : Outport
  wires:
  Build 4x4 Matrix1/1(A) -> M1/1
  Constant4/1 -> Build 4x4 Matrix1/1(A11)
  Gain3/1 -> Build 4x4 Matrix1/2(A21)
  Gain4/1 -> Build 4x4 Matrix1/4(A41)
  Gain5/1 -> Build 4x4 Matrix1/7(A32)
  Gain6/1 -> Build 4x4 Matrix1/8(A42)
  Constant3/1 -> Build 4x4 Matrix1/6(A22)
  Gain7/1 -> Build 4x4 Matrix1/9(A13)
  Constant2/1 -> Build 4x4 Matrix1/11(A33)
  Gain8/1 -> Build 4x4 Matrix1/12(A43)
  Demux1/1 -> Build 4x4 Matrix1/13(A14), Build 4x4 Matrix1/10(A23), Gain5/1, Gain4/1
  Demux1/3 -> Build 4x4 Matrix1/15(A34), Gain8/1, Gain3/1, Build 4x4 Matrix1/5(A12)
  Constant1/1 -> Build 4x4 Matrix1/16(A44)
  Demux1/2 -> Build 4x4 Matrix1/14(A24), Gain7/1, Build 4x4 Matrix1/3(A31), Gain6/1
  w/1 -> Demux1/1

== system desaturation/Attitude Determination and Non Linear Observer/Quaternion Integration /M2 ==
  q : Inport
  -q1^2+q2^2-q3^2+q4^2 : Subsystem
  -q1^2-q2^2+q3^2+q4^2 : Subsystem
  Add11 : Sum  Inputs=+-
  Add12 : Sum  Inputs=+-
  Add13 : Sum  Inputs=+-
  Add14 : Sum
  Add15 : Sum
  Add5 : Sum
  Build 3x3 Matrix1 : Subsystem
  Subsystem : Subsystem
  q1^2-q2^2-q3^2+q4^2 : Subsystem
  "M2 " : Outport
  wires:
  Build 3x3 Matrix1/1(A) -> "M2 "/1
  q1^2-q2^2-q3^2+q4^2/1(Out1) -> Build 3x3 Matrix1/1(A11)
  Add11/1 -> Build 3x3 Matrix1/2(A21)
  Add5/1 -> Build 3x3 Matrix1/3(A31)
  Add14/1 -> Build 3x3 Matrix1/4(A12)
  Add15/1 -> Build 3x3 Matrix1/8(A23)
  -q1^2+q2^2-q3^2+q4^2/1(Out1) -> Build 3x3 Matrix1/5(A22)
  Add13/1 -> Build 3x3 Matrix1/7("A13 ")
  Add12/1 -> Build 3x3 Matrix1/6(A32)
  -q1^2-q2^2+q3^2+q4^2/1(Out1) -> Build 3x3 Matrix1/9(A33)
  q/1 -> Subsystem/1(q), -q1^2+q2^2-q3^2+q4^2/1(q), -q1^2-q2^2+q3^2+q4^2/1(q), q1^2-q2^2-q3^2+q4^2/1(q)
  Subsystem/1(2q1q2) -> Add11/1, Add14/1
  Subsystem/2(2q1q3) -> Add5/1, Add13/1
  Subsystem/3(2q1q4) -> Add15/2, Add12/2
  Subsystem/6(2q3q4) -> Add11/2, Add14/2
  Subsystem/5(2q2q4) -> Add13/2, Add5/2
  Subsystem/4(2q2q3) -> Add15/1, Add12/1

== system desaturation/Attitude Determination and Non Linear Observer/Quaternion Integration /Normalization  ==
  "q " : Inport
  4D-Norm : Subsystem
  Divide : Product  Inputs=*/
  qNormalized : Outport
  wires:
  "q "/1 -> 4D-Norm/1(V), Divide/1
  4D-Norm/1(normV) -> Divide/2
  Divide/1 -> qNormalized/1

== system desaturation/Control and Actuators/Actuators/Cross Product ==
  a : Inport
  b : Inport  Port=2
  Add : Sum  Inputs=+-
  Add1 : Sum  Inputs=+-
  Add2 : Sum  Inputs=+-
  Demux : Demux  Outputs=3
  Demux1 : Demux  Outputs=3
  Product{,1..5} (6 alike) : Product
  Vector Concatenate : Concatenate  NumInputs=3
  c : Outport
  wires:
  Demux1/1 -> Product2/2, Product5/2  "Bx"
  Product2/1 -> Add1/1
  Vector Concatenate/1 -> c/1
  Add/1 -> Vector Concatenate/1
  Product3/1 -> Add1/2
  Product1/1 -> Add/2
  Product4/1 -> Add2/1
  Product/1 -> Add/1
  Demux/1 -> Product3/1, Product4/1  "Ax"
  Product5/1 -> Add2/2
  Demux/3 -> Product2/1, Product1/1  "Az"
  b/1 -> Demux1/1
  a/1 -> Demux/1
  Add2/1 -> Vector Concatenate/3
  Demux/2 -> Product5/1, Product/1  "Ay"
  Demux1/3 -> Product/2, Product3/2  "Bz"
  Demux1/2 -> Product4/2, Product1/2  "By"
  Add1/1 -> Vector Concatenate/2

== system desaturation/Control and Actuators/Actuators/Cross Product1 ==
  a : Inport
  b : Inport  Port=2
  Add : Sum  Inputs=+-
  Add1 : Sum  Inputs=+-
  Add2 : Sum  Inputs=+-
  Demux : Demux  Outputs=3
  Demux1 : Demux  Outputs=3
  Product{,1..5} (6 alike) : Product
  Vector Concatenate : Concatenate  NumInputs=3
  c : Outport
  wires:
  Demux1/1 -> Product2/2, Product5/2  "Bx"
  Product2/1 -> Add1/1
  Vector Concatenate/1 -> c/1
  Add/1 -> Vector Concatenate/1
  Product3/1 -> Add1/2
  Product1/1 -> Add/2
  Product4/1 -> Add2/1
  Product/1 -> Add/1
  Demux/1 -> Product3/1, Product4/1  "Ax"
  Product5/1 -> Add2/2
  Demux/3 -> Product2/1, Product1/1  "Az"
  b/1 -> Demux1/1
  a/1 -> Demux/1
  Add2/1 -> Vector Concatenate/3
  Demux/2 -> Product5/1, Product/1  "Ay"
  Demux1/3 -> Product/2, Product3/2  "Bz"
  Demux1/2 -> Product4/2, Product1/2  "By"
  Add1/1 -> Vector Concatenate/2

== system desaturation/Control and Actuators/Desaturation/3D Norm ==
  V : Inport
  Add : Sum  Inputs=+++
  Demux : Demux  Outputs=3
  Square : Math  Operator=square  SaturateOnIntegerOverflow=on
  Square Root : Sqrt  SaturateOnIntegerOverflow=on
  Square1 : Math  Operator=square  SaturateOnIntegerOverflow=on
  Square2 : Math  Operator=square  SaturateOnIntegerOverflow=on
  normV : Outport
  wires:
  Square Root/1 -> normV/1
  V/1 -> Demux/1
  Demux/3 -> Square2/1
  Square/1 -> Add/1
  Demux/1 -> Square/1
  Demux/2 -> Square1/1
  Square2/1 -> Add/3
  Square1/1 -> Add/2
  Add/1 -> Square Root/1

== system desaturation/Control and Actuators/Desaturation/Cross Product1 ==
  a : Inport
  b : Inport  Port=2
  Add : Sum  Inputs=+-
  Add1 : Sum  Inputs=+-
  Add2 : Sum  Inputs=+-
  Demux : Demux  Outputs=3
  Demux1 : Demux  Outputs=3
  Product{,1..5} (6 alike) : Product
  Vector Concatenate : Concatenate  NumInputs=3
  c : Outport
  wires:
  Demux1/1 -> Product2/2, Product5/2  "Bx"
  Product2/1 -> Add1/1
  Vector Concatenate/1 -> c/1
  Add/1 -> Vector Concatenate/1
  Product3/1 -> Add1/2
  Product1/1 -> Add/2
  Product4/1 -> Add2/1
  Product/1 -> Add/1
  Demux/1 -> Product3/1, Product4/1  "Ax"
  Product5/1 -> Add2/2
  Demux/3 -> Product2/1, Product1/1  "Az"
  b/1 -> Demux1/1
  a/1 -> Demux/1
  Add2/1 -> Vector Concatenate/3
  Demux/2 -> Product5/1, Product/1  "Ay"
  Demux1/3 -> Product/2, Product3/2  "Bz"
  Demux1/2 -> Product4/2, Product1/2  "By"
  Add1/1 -> Vector Concatenate/2

== system desaturation/Control and Actuators/Estimate Control Torque/Cross Product ==
  a : Inport
  b : Inport  Port=2
  Add : Sum  Inputs=+-
  Add1 : Sum  Inputs=+-
  Add2 : Sum  Inputs=+-
  Demux : Demux  Outputs=3
  Demux1 : Demux  Outputs=3
  Product{,1..5} (6 alike) : Product
  Vector Concatenate : Concatenate  NumInputs=3
  c : Outport
  wires:
  Demux1/1 -> Product2/2, Product5/2  "Bx"
  Product2/1 -> Add1/1
  Vector Concatenate/1 -> c/1
  Add/1 -> Vector Concatenate/1
  Product3/1 -> Add1/2
  Product1/1 -> Add/2
  Product4/1 -> Add2/1
  Product/1 -> Add/1
  Demux/1 -> Product3/1, Product4/1  "Ax"
  Product5/1 -> Add2/2
  Demux/3 -> Product2/1, Product1/1  "Az"
  b/1 -> Demux1/1
  a/1 -> Demux/1
  Add2/1 -> Vector Concatenate/3
  Demux/2 -> Product5/1, Product/1  "Ay"
  Demux1/3 -> Product/2, Product3/2  "Bz"
  Demux1/2 -> Product4/2, Product1/2  "By"
  Add1/1 -> Vector Concatenate/2

== system desaturation/Control and Actuators/Estimate Control Torque/Cross Product1 ==
  a : Inport
  b : Inport  Port=2
  Add : Sum  Inputs=+-
  Add1 : Sum  Inputs=+-
  Add2 : Sum  Inputs=+-
  Demux : Demux  Outputs=3
  Demux1 : Demux  Outputs=3
  Product{,1..5} (6 alike) : Product
  Vector Concatenate : Concatenate  NumInputs=3
  c : Outport
  wires:
  Demux1/1 -> Product2/2, Product5/2  "Bx"
  Product2/1 -> Add1/1
  Vector Concatenate/1 -> c/1
  Add/1 -> Vector Concatenate/1
  Product3/1 -> Add1/2
  Product1/1 -> Add/2
  Product4/1 -> Add2/1
  Product/1 -> Add/1
  Demux/1 -> Product3/1, Product4/1  "Ax"
  Product5/1 -> Add2/2
  Demux/3 -> Product2/1, Product1/1  "Az"
  b/1 -> Demux1/1
  a/1 -> Demux/1
  Add2/1 -> Vector Concatenate/3
  Demux/2 -> Product5/1, Product/1  "Ay"
  Demux1/3 -> Product/2, Product3/2  "Bz"
  Demux1/2 -> Product4/2, Product1/2  "By"
  Add1/1 -> Vector Concatenate/2

== system desaturation/Control and Actuators/Torque Allocation/3D Norm ==
  V : Inport
  Add : Sum  Inputs=+++
  Demux : Demux  Outputs=3
  Square : Math  Operator=square  SaturateOnIntegerOverflow=on
  Square Root : Sqrt  SaturateOnIntegerOverflow=on
  Square1 : Math  Operator=square  SaturateOnIntegerOverflow=on
  Square2 : Math  Operator=square  SaturateOnIntegerOverflow=on
  normV : Outport
  wires:
  Square Root/1 -> normV/1
  V/1 -> Demux/1
  Demux/3 -> Square2/1
  Square/1 -> Add/1
  Demux/1 -> Square/1
  Demux/2 -> Square1/1
  Square2/1 -> Add/3
  Square1/1 -> Add/2
  Add/1 -> Square Root/1

== system desaturation/Control and Actuators/Torque Allocation/Cross Product ==
  a : Inport
  b : Inport  Port=2
  Add : Sum  Inputs=+-
  Add1 : Sum  Inputs=+-
  Add2 : Sum  Inputs=+-
  Demux : Demux  Outputs=3
  Demux1 : Demux  Outputs=3
  Product{,1..5} (6 alike) : Product
  Vector Concatenate : Concatenate  NumInputs=3
  c : Outport
  wires:
  Demux1/1 -> Product2/2, Product5/2  "Bx"
  Product2/1 -> Add1/1
  Vector Concatenate/1 -> c/1
  Add/1 -> Vector Concatenate/1
  Product3/1 -> Add1/2
  Product1/1 -> Add/2
  Product4/1 -> Add2/1
  Product/1 -> Add/1
  Demux/1 -> Product3/1, Product4/1  "Ax"
  Product5/1 -> Add2/2
  Demux/3 -> Product2/1, Product1/1  "Az"
  b/1 -> Demux1/1
  a/1 -> Demux/1
  Add2/1 -> Vector Concatenate/3
  Demux/2 -> Product5/1, Product/1  "Ay"
  Demux1/3 -> Product/2, Product3/2  "Bz"
  Demux1/2 -> Product4/2, Product1/2  "By"
  Add1/1 -> Vector Concatenate/2

== system desaturation/Control and Actuators/Torque Allocation/Cross Product1 ==
  a : Inport
  b : Inport  Port=2
  Add : Sum  Inputs=+-
  Add1 : Sum  Inputs=+-
  Add2 : Sum  Inputs=+-
  Demux : Demux  Outputs=3
  Demux1 : Demux  Outputs=3
  Product{,1..5} (6 alike) : Product
  Vector Concatenate : Concatenate  NumInputs=3
  c : Outport
  wires:
  Demux1/1 -> Product2/2, Product5/2  "Bx"
  Product2/1 -> Add1/1
  Vector Concatenate/1 -> c/1
  Add/1 -> Vector Concatenate/1
  Product3/1 -> Add1/2
  Product1/1 -> Add/2
  Product4/1 -> Add2/1
  Product/1 -> Add/1
  Demux/1 -> Product3/1, Product4/1  "Ax"
  Product5/1 -> Add2/2
  Demux/3 -> Product2/1, Product1/1  "Az"
  b/1 -> Demux1/1
  a/1 -> Demux/1
  Add2/1 -> Vector Concatenate/3
  Demux/2 -> Product5/1, Product/1  "Ay"
  Demux1/3 -> Product/2, Product3/2  "Bz"
  Demux1/2 -> Product4/2, Product1/2  "By"
  Add1/1 -> Vector Concatenate/2

== system desaturation/Environment/Earth's Shadow/3D Norm ==
  V : Inport
  Add : Sum  Inputs=+++
  Demux : Demux  Outputs=3
  Square : Math  Operator=square  SaturateOnIntegerOverflow=on
  Square Root : Sqrt  SaturateOnIntegerOverflow=on
  Square1 : Math  Operator=square  SaturateOnIntegerOverflow=on
  Square2 : Math  Operator=square  SaturateOnIntegerOverflow=on
  normV : Outport
  wires:
  Square Root/1 -> normV/1
  V/1 -> Demux/1
  Demux/3 -> Square2/1
  Square/1 -> Add/1
  Demux/1 -> Square/1
  Demux/2 -> Square1/1
  Square2/1 -> Add/3
  Square1/1 -> Add/2
  Add/1 -> Square Root/1

== system desaturation/Environment/Gravity Gradient Torque/3D-Norm ==
  V : Inport
  Add : Sum  Inputs=+++
  Demux : Demux  Outputs=3
  Square : Math  Operator=square  SaturateOnIntegerOverflow=on
  Square Root : Sqrt  SaturateOnIntegerOverflow=on
  Square1 : Math  Operator=square  SaturateOnIntegerOverflow=on
  Square2 : Math  Operator=square  SaturateOnIntegerOverflow=on
  normV : Outport
  wires:
  Square Root/1 -> normV/1
  Add/1 -> Square Root/1
  Square2/1 -> Add/3
  Square1/1 -> Add/2
  Square/1 -> Add/1
  Demux/1 -> Square/1
  Demux/2 -> Square1/1
  Demux/3 -> Square2/1
  V/1 -> Demux/1

== system desaturation/Environment/Magnetic Torque/Cross Product ==
  a : Inport
  b : Inport  Port=2
  Add : Sum  Inputs=+-
  Add1 : Sum  Inputs=+-
  Add2 : Sum  Inputs=+-
  Demux : Demux  Outputs=3
  Demux1 : Demux  Outputs=3
  Product{,1..5} (6 alike) : Product
  Vector Concatenate : Concatenate  NumInputs=3
  c : Outport
  wires:
  Demux1/1 -> Product2/2, Product5/2  "Bx"
  Product2/1 -> Add1/1
  Vector Concatenate/1 -> c/1
  Add/1 -> Vector Concatenate/1
  Product3/1 -> Add1/2
  Product1/1 -> Add/2
  Product4/1 -> Add2/1
  Product/1 -> Add/1
  Demux/1 -> Product3/1, Product4/1  "Ax"
  Product5/1 -> Add2/2
  Demux/3 -> Product2/1, Product1/1  "Az"
  b/1 -> Demux1/1
  a/1 -> Demux/1
  Add2/1 -> Vector Concatenate/3
  Demux/2 -> Product5/1, Product/1  "Ay"
  Demux1/3 -> Product/2, Product3/2  "Bz"
  Demux1/2 -> Product4/2, Product1/2  "By"
  Add1/1 -> Vector Concatenate/2

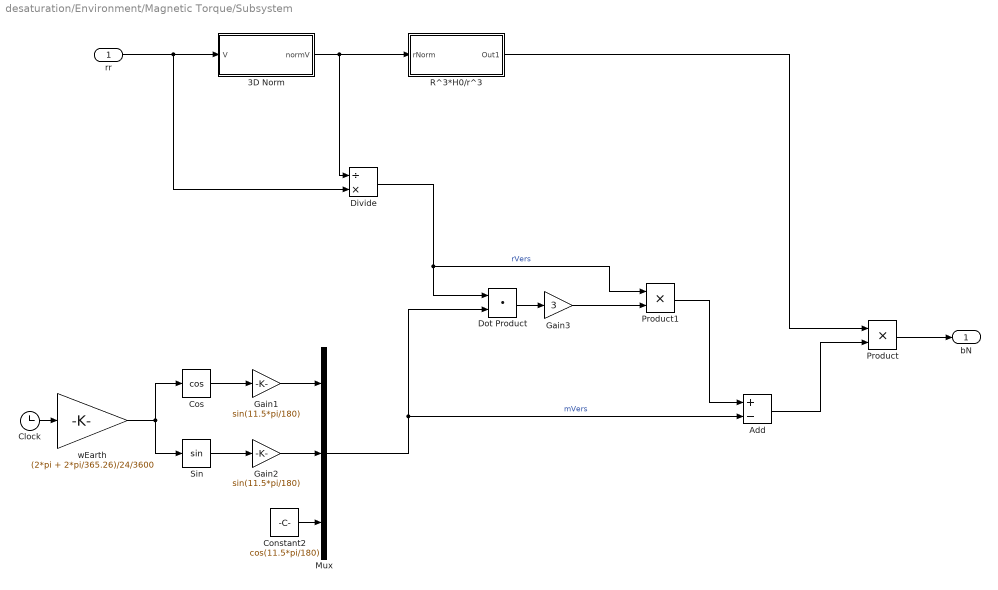
== system desaturation/Environment/Magnetic Torque/Subsystem ==
  rr : Inport
  3D Norm : Subsystem
  Add : Sum  Inputs=+-
  Clock : Clock
  Constant2 : Constant  Value=cos(11.5*pi/180)
  Cos : Trigonometry  Operator=cos
  Divide : Product  Inputs=/*
  Dot Product : DotProduct  InputSameDT=on  OutDataTypeStr=Inherit: Inherit via internal rule
  Gain1 : Gain  Gain=sin(11.5*pi/180)
  Gain2 : Gain  Gain=sin(11.5*pi/180)
  Gain3 : Gain  Gain=3
  Mux : Mux  Inputs=3
  Product : Product
  Product1 : Product
  R^3*H0/r^3 : Subsystem
  Sin : Trigonometry
  wEarth : Gain  Gain=(2*pi + 2*pi/365.26)/24/3600
  bN : Outport
  wires:
  3D Norm/1(normV) -> Divide/1, R^3*H0/r^3/1(rNorm)
  Cos/1 -> Gain1/1
  Sin/1 -> Gain2/1
  Gain2/1 -> Mux/2
  rr/1 -> 3D Norm/1(V), Divide/2
  Product1/1 -> Add/1
  wEarth/1 -> Sin/1, Cos/1
  Constant2/1 -> Mux/3
  Gain1/1 -> Mux/1
  Gain3/1 -> Product1/2
  Product/1 -> bN/1
  Add/1 -> Product/2
  Clock/1 -> wEarth/1
  R^3*H0/r^3/1(Out1) -> Product/1
  Dot Product/1 -> Gain3/1
  Divide/1 -> Product1/1, Dot Product/1  "rVers"
  Mux/1 -> Dot Product/2, Add/2  "mVers"

== system desaturation/Environment/Unperturbed Orbit/Subsystem ==
  theta : Inport
  Add : Sum
  Constant : Constant
  Cos : Trigonometry  Operator=cos
  Gain : Gain  Gain=data.orbit.e
  Gain1 : Gain  Gain=data.orbit.n/(1-data.orbit.e^2)^(3/2)
  Square : Math  Operator=square  SaturateOnIntegerOverflow=on
  theta_dot : Outport
  wires:
  theta/1 -> Cos/1
  Cos/1 -> Gain/1
  Gain/1 -> Add/1
  Constant/1 -> Add/2
  Add/1 -> Square/1
  Square/1 -> Gain1/1
  Gain1/1 -> theta_dot/1

== system desaturation/Environment/Unperturbed Orbit/Subsystem1 ==
  theta : Inport
  Build 3x3 Matrix : Subsystem
  Constant : Constant  Value=0
  Constant1 : Constant
  Cos1 : Trigonometry  Operator=cos
  Cos2 : Trigonometry  Operator=cos
  Gain : Gain  Gain=-1
  Gain1 : Gain  Gain=[1 0 0; 0 cos(data.orbit.i) sin(data.orbit.i); 0 -sin(data.orbit.i) cos(data.orbit.i)]  Multiplication=Matrix(u*K)
  Sin : Trigonometry
  Sin1 : Trigonometry
  ALN : Outport
  wires:
  Cos1/1 -> Build 3x3 Matrix/1(A11)
  theta/1 -> Cos2/1, Sin1/1, Cos1/1, Sin/1
  Sin/1 -> Gain/1
  Gain/1 -> Build 3x3 Matrix/2(A21)
  Sin1/1 -> Build 3x3 Matrix/4(A12)
  Cos2/1 -> Build 3x3 Matrix/5(A22)
  Constant/1 -> Build 3x3 Matrix/8(A23), Build 3x3 Matrix/7("A13 "), Build 3x3 Matrix/6(A32), Build 3x3 Matrix/3(A31)
  Constant1/1 -> Build 3x3 Matrix/9(A33)
  Build 3x3 Matrix/1(A) -> Gain1/1
  Gain1/1 -> ALN/1

== system desaturation/Environment/Unperturbed Orbit/Subsystem2 ==
  theta : Inport
  Add : Sum
  Constant : Constant
  Constant1 : Constant  Value=data.orbit.a*(1-data.orbit.e^2)
  Cos : Trigonometry  Operator=cos
  Cos1 : Trigonometry  Operator=cos
  Divide : Product  Inputs=/*
  Gain : Gain  Gain=cos(data.orbit.i)
  Gain1 : Gain  Gain=sin(data.orbit.i)
  Gain3 : Gain  Gain=data.orbit.e
  Mux : Mux  Inputs=3
  Product : Product
  Sin : Trigonometry
  Sin1 : Trigonometry
  rr : Outport
  wires:
  Cos/1 -> Mux/1
  theta/1 -> Cos1/1, Sin1/1, Cos/1, Sin/1
  Gain/1 -> Mux/2
  Gain1/1 -> Mux/3
  Sin/1 -> Gain/1
  Sin1/1 -> Gain1/1
  Cos1/1 -> Gain3/1
  Gain3/1 -> Add/1
  Constant/1 -> Add/2
  Add/1 -> Divide/1
  Constant1/1 -> Divide/2
  Divide/1 -> Product/2
  Mux/1 -> Product/1
  Product/1 -> rr/1

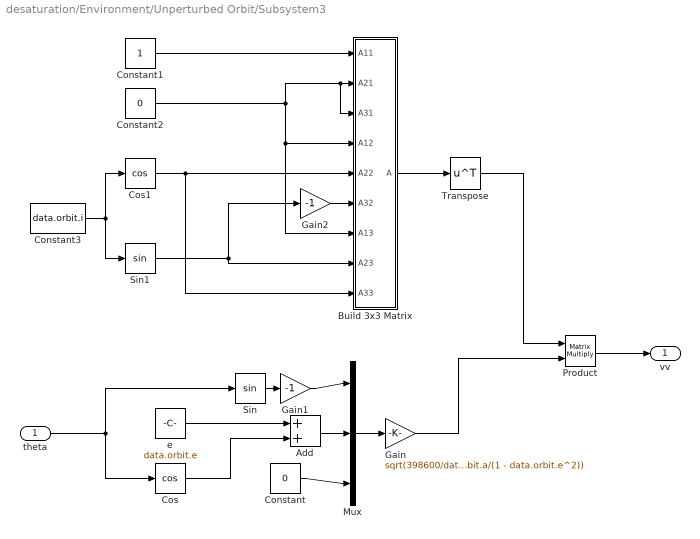
== system desaturation/Environment/Unperturbed Orbit/Subsystem3 ==
  theta : Inport
  Add : Sum
  Build 3x3 Matrix : Subsystem
  Constant : Constant  Value=0
  Constant1 : Constant
  Constant2 : Constant  Value=0
  Constant3 : Constant  Value=data.orbit.i
  Cos : Trigonometry  Operator=cos
  Cos1 : Trigonometry  Operator=cos
  Gain : Gain  Gain=sqrt(398600/data.orbit.a/(1 - data.orbit.e^2))
  Gain1 : Gain  Gain=-1
  Gain2 : Gain  Gain=-1
  Mux : Mux  Inputs=3
  Product : Product  Multiplication=Matrix(*)
  Sin : Trigonometry
  Sin1 : Trigonometry
  Transpose : Math  Operator=transpose  SaturateOnIntegerOverflow=on
  e : Constant  Value=data.orbit.e
  vv : Outport
  wires:
  Mux/1 -> Gain/1
  theta/1 -> Cos/1, Sin/1
  Constant/1 -> Mux/3
  Add/1 -> Mux/2
  Cos/1 -> Add/2
  Sin/1 -> Gain1/1
  e/1 -> Add/1
  Gain1/1 -> Mux/1
  Constant3/1 -> Sin1/1, Cos1/1
  Constant1/1 -> Build 3x3 Matrix/1(A11)
  Constant2/1 -> Build 3x3 Matrix/3(A31), Build 3x3 Matrix/2(A21), Build 3x3 Matrix/4(A12), Build 3x3 Matrix/7("A13 ")
  Cos1/1 -> Build 3x3 Matrix/9(A33), Build 3x3 Matrix/5(A22)
  Gain2/1 -> Build 3x3 Matrix/6(A32)
  Sin1/1 -> Build 3x3 Matrix/8(A23), Gain2/1
  Build 3x3 Matrix/1(A) -> Transpose/1
  Transpose/1 -> Product/1
  Gain/1 -> Product/2
  Product/1 -> vv/1

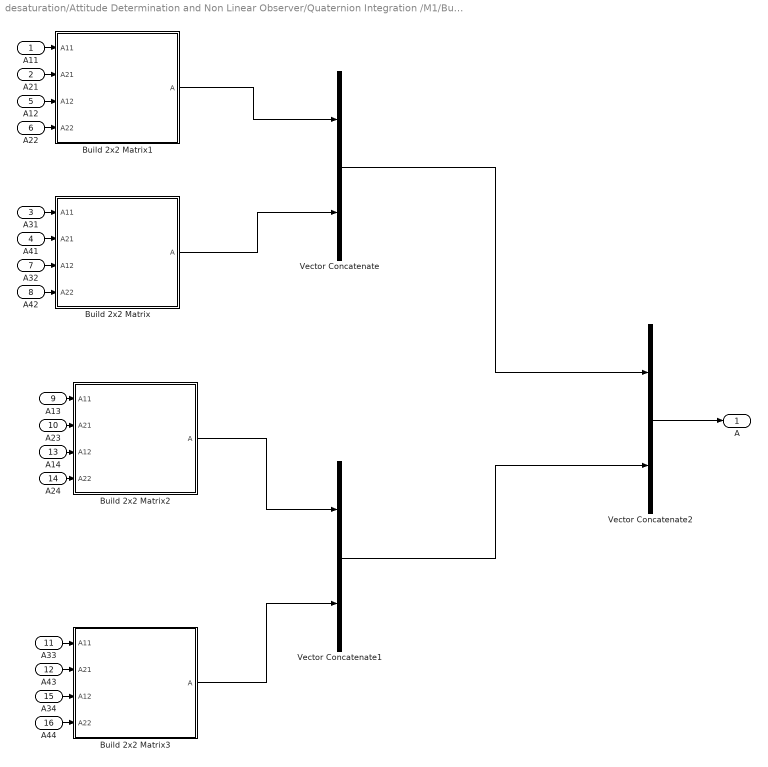
== system desaturation/Attitude Determination and Non Linear Observer/Quaternion Integration /M1/Build 4x4 Matrix1 ==
  A11 : Inport
  A21 : Inport  Port=2
  A31 : Inport  Port=3
  A41 : Inport  Port=4
  A12 : Inport  Port=5
  A22 : Inport  Port=6
  A32 : Inport  Port=7
  A42 : Inport  Port=8
  A13 : Inport  Port=9
  A23 : Inport  Port=10
  A33 : Inport  Port=11
  A43 : Inport  Port=12
  A14 : Inport  Port=13
  A24 : Inport  Port=14
  A34 : Inport  Port=15
  A44 : Inport  Port=16
  Build 2x2 Matrix : Subsystem
  Build 2x2 Matrix1 : Subsystem
  Build 2x2 Matrix2 : Subsystem
  Build 2x2 Matrix3 : Subsystem
  Vector Concatenate : Concatenate  Mode=Multidimensional array
  Vector Concatenate1 : Concatenate  Mode=Multidimensional array
  Vector Concatenate2 : Concatenate  Mode=Multidimensional array  ConcatenateDimension=2
  A : Outport
  wires:
  Build 2x2 Matrix2/1(A) -> Vector Concatenate1/1
  Build 2x2 Matrix3/1(A) -> Vector Concatenate1/2
  Vector Concatenate2/1 -> A/1
  Vector Concatenate1/1 -> Vector Concatenate2/2
  Vector Concatenate/1 -> Vector Concatenate2/1
  Build 2x2 Matrix/1(A) -> Vector Concatenate/2
  Build 2x2 Matrix1/1(A) -> Vector Concatenate/1
  A44/1 -> Build 2x2 Matrix3/4(A22)
  A34/1 -> Build 2x2 Matrix3/3(A12)
  A43/1 -> Build 2x2 Matrix3/2(A21)
  A33/1 -> Build 2x2 Matrix3/1(A11)
  A42/1 -> Build 2x2 Matrix/4(A22)
  A32/1 -> Build 2x2 Matrix/3(A12)
  A41/1 -> Build 2x2 Matrix/2(A21)
  A31/1 -> Build 2x2 Matrix/1(A11)
  A24/1 -> Build 2x2 Matrix2/4(A22)
  A14/1 -> Build 2x2 Matrix2/3(A12)
  A23/1 -> Build 2x2 Matrix2/2(A21)
  A13/1 -> Build 2x2 Matrix2/1(A11)
  A22/1 -> Build 2x2 Matrix1/4(A22)
  A12/1 -> Build 2x2 Matrix1/3(A12)
  A21/1 -> Build 2x2 Matrix1/2(A21)
  A11/1 -> Build 2x2 Matrix1/1(A11)

== system desaturation/Attitude Determination and Non Linear Observer/Quaternion Integration /M2/-q1^2+q2^2-q3^2+q4^2 ==
  q : Inport
  Add : Sum  Inputs=-+-+
  Demux : Demux
  Square{,1..3} (4 alike) : Math  Operator=square  SaturateOnIntegerOverflow=on
  Out1 : Outport
  wires:
  q/1 -> Demux/1
  Demux/1 -> Square/1
  Demux/2 -> Square1/1
  Demux/3 -> Square2/1
  Demux/4 -> Square3/1
  Add/1 -> Out1/1
  Square/1 -> Add/1
  Square1/1 -> Add/2
  Square2/1 -> Add/3
  Square3/1 -> Add/4

== system desaturation/Attitude Determination and Non Linear Observer/Quaternion Integration /M2/-q1^2-q2^2+q3^2+q4^2 ==
  q : Inport
  Add : Sum  Inputs=--++
  Demux : Demux
  Square{,1..3} (4 alike) : Math  Operator=square  SaturateOnIntegerOverflow=on
  Out1 : Outport
  wires:
  q/1 -> Demux/1
  Demux/1 -> Square/1
  Demux/2 -> Square1/1
  Demux/3 -> Square2/1
  Demux/4 -> Square3/1
  Add/1 -> Out1/1
  Square/1 -> Add/1
  Square1/1 -> Add/2
  Square2/1 -> Add/3
  Square3/1 -> Add/4

== system desaturation/Attitude Determination and Non Linear Observer/Quaternion Integration /M2/Build 3x3 Matrix1 ==
  A11 : Inport
  A21 : Inport  Port=2
  A31 : Inport  Port=3
  A12 : Inport  Port=4
  A22 : Inport  Port=5
  A32 : Inport  Port=6
  "A13 " : Inport  Port=7
  A23 : Inport  Port=8
  A33 : Inport  Port=9
  Mux : Mux  Inputs=3
  Mux1 : Mux  Inputs=3
  Mux2 : Mux  Inputs=3
  Vector Concatenate : Concatenate  NumInputs=3  Mode=Multidimensional array  ConcatenateDimension=2
  A : Outport
  wires:
  Vector Concatenate/1 -> A/1
  Mux2/1 -> Vector Concatenate/3
  Mux1/1 -> Vector Concatenate/2
  Mux/1 -> Vector Concatenate/1
  A33/1 -> Mux2/3
  A23/1 -> Mux2/2
  "A13 "/1 -> Mux2/1
  A32/1 -> Mux1/3
  A22/1 -> Mux1/2
  A12/1 -> Mux1/1
  A31/1 -> Mux/3
  A21/1 -> Mux/2
  A11/1 -> Mux/1
